simulink library "FuelSystemLibrary"  (R2014b)
settings: Solver=ode45  SolverMode=SingleTasking  StartTime=0.0  StopTime=10.0  RelTol=1e-3
undefined symbols (not defined in the file): BooleanOff, BooleanOn, BoolThreshold, BowserOnPressure, CouplingOffPressure, CouplingOnPressure, DefaultTemp, DiffuserResistance, DiscreteSwitchOff, DiscreteSwitchOn, DiscreteSwitchThreshold, FloatingPressure, FlowNoOverride, FspSamplingPeriod, FuelSpecificHeatCapacity, g, InfiniteFlow, InfiniteMass, InfiniteResistance, InfiniteTime, InfiniteVolume, kpl2kpm3, MaxAValue, MaxBValue, MeterNoReset, MinAValue, MinBValue, NearZeroMass, NearZeroTime, NoError, NominalAValue, NominalBValue, NonRetResistance, NoReset, NullBasePress, PerCycle2PerSec, PerSec2PerCycle, PipeDisconnected, PipeResistance, PumpOnTime, TankFixedMassError, TankInletResistance, TankInstPortStartOffset, TankNoReset, TypicalFuelDensity, ValveClosedPosition, ValveOnResistance, ValveOpenPosition, ValveOpenTime
libraries: FuelSystemLibrary x251, WrightSolverLib x50, simulink x1
(part 3 of 4)

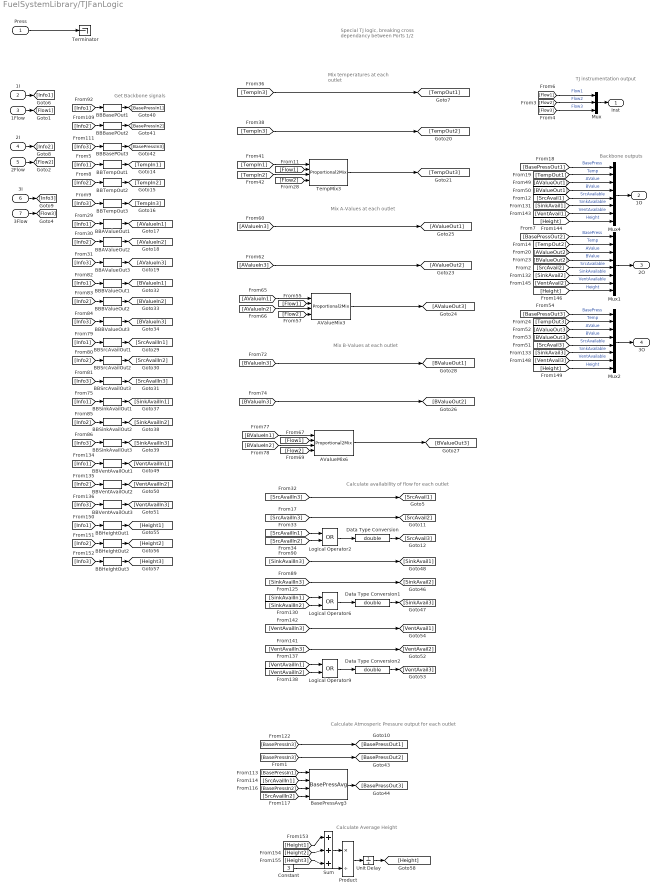
== system FuelSystemLibrary/TJFanLogic ==
  note: TJ instrumentation
      |  output
  note: Calculate availability of flow for each outlet
  note: Mix temperatures
      | at each outlet
  note: Backbone outputs
  note: Get Backbone signals
  note: Mix A-Values at each outlet
  note: Mix B-Values at each outlet
  note: Calculate Atmosperic Pressure output for each outlet
  note: Special TJ logic, breaking
      | cross dependancy
      | between Ports 1/2
  note: Calculate Average Height
  Press : Inport
  1I : Inport  Port=2
  1Flow : Inport  Port=3
  2I : Inport  Port=4
  2Flow : Inport  Port=5
  3I : Inport  Port=6
  3Flow : Inport  Port=7
  AValueMix3 : FuelSystemLibrary/Proportional2Mix
  AValueMix6 : FuelSystemLibrary/Proportional2Mix
  BBAValueOut1 : FuelSystemLibrary/BBAValueOut
  BBAValueOut2 : FuelSystemLibrary/BBAValueOut
  BBAValueOut3 : FuelSystemLibrary/BBAValueOut
  BBBValueOut1 : FuelSystemLibrary/BBBValueOut
  BBBValueOut2 : FuelSystemLibrary/BBBValueOut
  BBBValueOut3 : FuelSystemLibrary/BBBValueOut
  BBBasePOut1 : FuelSystemLibrary/BBBasePOut
  BBBasePOut2 : FuelSystemLibrary/BBBasePOut
  BBBasePOut3 : FuelSystemLibrary/BBBasePOut
  BBHeightOut1 : FuelSystemLibrary/BBHeightOut
  BBHeightOut2 : FuelSystemLibrary/BBHeightOut
  BBHeightOut3 : FuelSystemLibrary/BBHeightOut
  BBSinkAvailOut1 : FuelSystemLibrary/BBSinkAvailOut
  BBSinkAvailOut2 : FuelSystemLibrary/BBSinkAvailOut
  BBSinkAvailOut3 : FuelSystemLibrary/BBSinkAvailOut
  BBSrcAvailOut1 : FuelSystemLibrary/BBSrcAvailOut
  BBSrcAvailOut2 : FuelSystemLibrary/BBSrcAvailOut
  BBSrcAvailOut3 : FuelSystemLibrary/BBSrcAvailOut
  BBTempOut1 : FuelSystemLibrary/BBTempOut
  BBTempOut2 : FuelSystemLibrary/BBTempOut
  BBTempOut3 : FuelSystemLibrary/BBTempOut
  BBVentAvailOut1 : FuelSystemLibrary/BBVentAvailOut
  BBVentAvailOut2 : FuelSystemLibrary/BBVentAvailOut
  BBVentAvailOut3 : FuelSystemLibrary/BBVentAvailOut
  BasePressAvg3 : FuelSystemLibrary/BasePressAvg
  Constant : Constant  Value=3
  Data Type Conversion : DataTypeConversion  OutDataTypeStr=double
  Data Type Conversion1 : DataTypeConversion  OutDataTypeStr=double
  Data Type Conversion2 : DataTypeConversion  OutDataTypeStr=double
  Logical Operator2 : Logic  Operator=OR  AllPortsSameDT=off
  Logical Operator6 : Logic  Operator=OR  AllPortsSameDT=off
  Logical Operator9 : Logic  Operator=OR  AllPortsSameDT=off
  Mux : Mux  Inputs=[1 1 1]
  Mux1 : Mux  Inputs=8
  Mux2 : Mux  Inputs=8
  Mux4 : Mux  Inputs=8
  Product : Product  Inputs=*/  SaturateOnIntegerOverflow=on  InputSameDT=on  OutDataTypeStr=Inherit: Same as first input
  Sum : Sum  Inputs=|+++  SaturateOnIntegerOverflow=on  InputSameDT=on  OutDataTypeStr=Inherit: Same as first input
  TempMix3 : FuelSystemLibrary/Proportional2Mix
  Terminator : Terminator
  Unit Delay : UnitDelay  SampleTime=FspSamplingPeriod
  Inst : Outport
  1O : Outport  Port=2
  2O : Outport  Port=3
  3O : Outport  Port=4
  wires:
  1I/1 -> [Info1]
  1Flow/1 -> [Flow1]
  2Flow/1 -> [Flow2]
  3I/1 -> [Info3]
  3Flow/1 -> [Flow3]
  2I/1 -> [Info2]
  [Flow2] -> Mux/2  "Flow2"
  [Flow1] -> Mux/1  "Flow1"
  [Flow3] -> Mux/3  "Flow3"
  [Info1] -> BBTempOut1/1
  [Info2] -> BBTempOut2/1
  [Info3] -> BBTempOut3/1
  [Flow2] -> TempMix3/4
  BBTempOut1/1 -> [TempIn1]
  BBTempOut2/1 -> [TempIn2]
  BBTempOut3/1 -> [TempIn3]
  [Info1] -> BBAValueOut1/1
  [Info2] -> BBAValueOut2/1
  [Info3] -> BBAValueOut3/1
  [SrcAvailIn3] -> [SrcAvail1]
  [SrcAvailIn3] -> [SrcAvail2]
  [SrcAvailIn1] -> Logical Operator2/1
  [SrcAvailIn2] -> Logical Operator2/2
  Logical Operator2/1 -> Data Type Conversion/1
  [TempIn3] -> [TempOut1]
  [TempIn3] -> [TempOut2]
  [TempIn1] -> TempMix3/1
  [TempIn2] -> TempMix3/3
  [Flow1] -> TempMix3/2
  [SrcAvail1] -> Mux4/5  "SrcAvailable"
  [TempOut1] -> Mux4/2  "Temp"
  [BasePressOut1] -> Mux4/1  "BasePress"
  [AValueOut1] -> Mux4/3  "AValue"
  [BValueOut1] -> Mux4/4  "BValue"
  Mux4/1 -> 1O/1
  [SrcAvail2] -> Mux1/5  "SrcAvailable"
  [TempOut2] -> Mux1/2  "Temp"
  [BasePressOut2] -> Mux1/1  "BasePress"
  [AValueOut2] -> Mux1/3  "AValue"
  [BValueOut2] -> Mux1/4  "BValue"
  Mux1/1 -> 2O/1
  [SrcAvail3] -> Mux2/5  "SrcAvailable"
  [TempOut3] -> Mux2/2  "Temp"
  [BasePressOut3] -> Mux2/1  "BasePress"
  [AValueOut3] -> Mux2/3  "AValue"
  [BValueOut3] -> Mux2/4  "BValue"
  [Flow2] -> AValueMix3/4
  [AValueIn3] -> [AValueOut1]
  [AValueIn3] -> [AValueOut2]
  [AValueIn1] -> AValueMix3/1
  [AValueIn2] -> AValueMix3/3
  AValueMix3/1 -> [AValueOut3]
  [Flow1] -> AValueMix3/2
  [Flow2] -> AValueMix6/4
  [BValueIn3] -> [BValueOut1]
  [BValueIn3] -> [BValueOut2]
  [BValueIn1] -> AValueMix6/1
  [BValueIn2] -> AValueMix6/3
  AValueMix6/1 -> [BValueOut3]
  [Flow1] -> AValueMix6/2
  [Info1] -> BBSrcAvailOut1/1
  [Info2] -> BBSrcAvailOut2/1
  [Info3] -> BBSrcAvailOut3/1
  BBSrcAvailOut1/1 -> [SrcAvailIn1]
  BBSrcAvailOut2/1 -> [SrcAvailIn2]
  BBSrcAvailOut3/1 -> [SrcAvailIn3]
  BBAValueOut1/1 -> [AValueIn1]
  BBAValueOut2/1 -> [AValueIn2]
  BBAValueOut3/1 -> [AValueIn3]
  [Info1] -> BBBValueOut1/1
  [Info2] -> BBBValueOut2/1
  [Info3] -> BBBValueOut3/1
  BBBValueOut1/1 -> [BValueIn1]
  BBBValueOut2/1 -> [BValueIn2]
  BBBValueOut3/1 -> [BValueIn3]
  TempMix3/1 -> [TempOut3]
  Press/1 -> Terminator/1
  [Info1] -> BBBasePOut1/1
  BBBasePOut1/1 -> [BasePressIn1]
  [Info2] -> BBBasePOut2/1
  [Info3] -> BBBasePOut3/1
  BBBasePOut2/1 -> [BasePressIn2]
  BBBasePOut3/1 -> [BasePressIn3]
  [BasePressIn3] -> [BasePressOut1]
  [BasePressIn3] -> [BasePressOut2]
  [BasePressIn1] -> BasePressAvg3/1
  [SrcAvailIn1] -> BasePressAvg3/2
  [BasePressIn2] -> BasePressAvg3/3
  [SrcAvailIn2] -> BasePressAvg3/4
  BasePressAvg3/1 -> [BasePressOut3]
  [Info1] -> BBSinkAvailOut1/1
  BBSinkAvailOut1/1 -> [SinkAvailIn1]
  [Info2] -> BBSinkAvailOut2/1
  BBSinkAvailOut2/1 -> [SinkAvailIn2]
  [Info3] -> BBSinkAvailOut3/1
  BBSinkAvailOut3/1 -> [SinkAvailIn3]
  [SinkAvailIn3] -> [SinkAvail1]
  [SinkAvailIn3] -> [SinkAvail2]
  [SinkAvailIn1] -> Logical Operator6/1
  [SinkAvailIn2] -> Logical Operator6/2
  Logical Operator6/1 -> Data Type Conversion1/1
  [SinkAvail1] -> Mux4/6  "SinkAvailable"
  [SinkAvail2] -> Mux1/6  "SinkAvailable"
  [SinkAvail3] -> Mux2/6  "SinkAvailable"
  [Info1] -> BBVentAvailOut1/1
  BBVentAvailOut1/1 -> [VentAvailIn1]
  [Info2] -> BBVentAvailOut2/1
  BBVentAvailOut2/1 -> [VentAvailIn2]
  [Info3] -> BBVentAvailOut3/1
  BBVentAvailOut3/1 -> [VentAvailIn3]
  [VentAvailIn3] -> [VentAvail1]
  [VentAvailIn3] -> [VentAvail2]
  [VentAvailIn1] -> Logical Operator9/1
  [VentAvailIn2] -> Logical Operator9/2
  Logical Operator9/1 -> Data Type Conversion2/1
  [VentAvail1] -> Mux4/7  "VentAvailable"
  [Height] -> Mux4/8  "Height"
  [VentAvail2] -> Mux1/7  "VentAvailable"
  [Height] -> Mux1/8  "Height"
  Mux2/1 -> 3O/1
  [VentAvail3] -> Mux2/7  "VentAvailable"
  [Height] -> Mux2/8  "Height"
  [Info1] -> BBHeightOut1/1
  BBHeightOut1/1 -> [Height1]
  [Info2] -> BBHeightOut2/1
  BBHeightOut2/1 -> [Height2]
  [Info3] -> BBHeightOut3/1
  BBHeightOut3/1 -> [Height3]
  Mux/1 -> Inst/1
  Data Type Conversion/1 -> [SrcAvail3]
  Data Type Conversion1/1 -> [SinkAvail3]
  Data Type Conversion2/1 -> [VentAvail3]
  [Height1] -> Sum/1
  [Height2] -> Sum/2
  [Height3] -> Sum/3
  Sum/1 -> Product/1
  Product/1 -> Unit Delay/1
  Constant/1 -> Product/2
  Unit Delay/1 -> [Height]

== system FuelSystemLibrary/TJIntersect ==
  note: TJNet2I10 - Block to model T-junction behaviour - currently "perfect" connection
      |
      | Revision History -
      | Issue 1.0 - ?? - SW - Initial Issue
      | Issue 1.1 - 28th October 2005 - DR - Added to FSP Generic Library
  TJ : WrightSolverLib/TJ
  1P : PMIOPort  Tag=PMCPort  Port=1  Side=Left
  2P : PMIOPort  Tag=PMCPort  Port=2  Side=Left
  3P : PMIOPort  Tag=PMCPort  Port=3  Side=Right
  connections:
  1P/RConn1 -- TJ/LConn1
  TJ/RConn1 -- 3P/RConn1
  2P/RConn1 -- TJ/RConn2

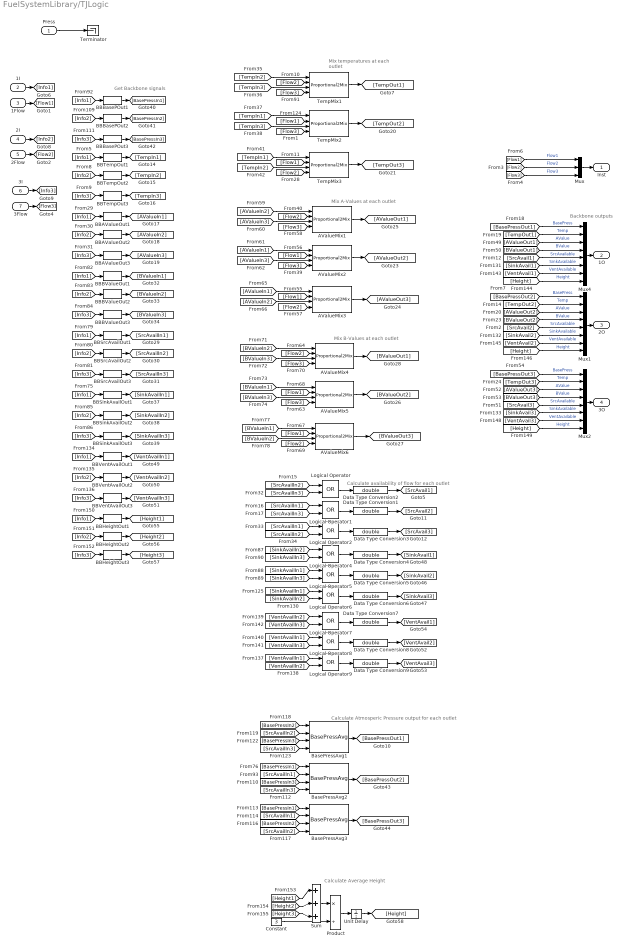
== system FuelSystemLibrary/TJLogic ==
  note: Backbone outputs
  note: Get Backbone signals
  note: Calculate Average Height
  note: Mix B-Values at each outlet
  note: Mix A-Values at each outlet
  note: Mix temperatures
      | at each outlet
  note: Calculate availability of flow for each outlet
  note: Calculate Atmosperic Pressure output for each outlet
  Press : Inport
  1I : Inport  Port=2
  1Flow : Inport  Port=3
  2I : Inport  Port=4
  2Flow : Inport  Port=5
  3I : Inport  Port=6
  3Flow : Inport  Port=7
  AValueMix{1..6} (6 alike) : FuelSystemLibrary/Proportional2Mix
  BBAValueOut1 : FuelSystemLibrary/BBAValueOut
  BBAValueOut2 : FuelSystemLibrary/BBAValueOut
  BBAValueOut3 : FuelSystemLibrary/BBAValueOut
  BBBValueOut1 : FuelSystemLibrary/BBBValueOut
  BBBValueOut2 : FuelSystemLibrary/BBBValueOut
  BBBValueOut3 : FuelSystemLibrary/BBBValueOut
  BBBasePOut1 : FuelSystemLibrary/BBBasePOut
  BBBasePOut2 : FuelSystemLibrary/BBBasePOut
  BBBasePOut3 : FuelSystemLibrary/BBBasePOut
  BBHeightOut1 : FuelSystemLibrary/BBHeightOut
  BBHeightOut2 : FuelSystemLibrary/BBHeightOut
  BBHeightOut3 : FuelSystemLibrary/BBHeightOut
  BBSinkAvailOut1 : FuelSystemLibrary/BBSinkAvailOut
  BBSinkAvailOut2 : FuelSystemLibrary/BBSinkAvailOut
  BBSinkAvailOut3 : FuelSystemLibrary/BBSinkAvailOut
  BBSrcAvailOut1 : FuelSystemLibrary/BBSrcAvailOut
  BBSrcAvailOut2 : FuelSystemLibrary/BBSrcAvailOut
  BBSrcAvailOut3 : FuelSystemLibrary/BBSrcAvailOut
  BBTempOut1 : FuelSystemLibrary/BBTempOut
  BBTempOut2 : FuelSystemLibrary/BBTempOut
  BBTempOut3 : FuelSystemLibrary/BBTempOut
  BBVentAvailOut1 : FuelSystemLibrary/BBVentAvailOut
  BBVentAvailOut2 : FuelSystemLibrary/BBVentAvailOut
  BBVentAvailOut3 : FuelSystemLibrary/BBVentAvailOut
  BasePressAvg1 : FuelSystemLibrary/BasePressAvg
  BasePressAvg2 : FuelSystemLibrary/BasePressAvg
  BasePressAvg3 : FuelSystemLibrary/BasePressAvg
  Constant : Constant  Value=3
  Data Type Conversion{1..9} (9 alike) : DataTypeConversion  OutDataTypeStr=double
  Logical Operator{,1..2,4..9} (9 alike) : Logic  Operator=OR  AllPortsSameDT=off
  Mux : Mux  Inputs=[1 1 1]
  Mux1 : Mux  Inputs=8
  Mux2 : Mux  Inputs=8
  Mux4 : Mux  Inputs=8
  Product : Product  Inputs=*/  SaturateOnIntegerOverflow=on  InputSameDT=on  OutDataTypeStr=Inherit: Same as first input
  Sum : Sum  Inputs=|+++  SaturateOnIntegerOverflow=on  InputSameDT=on  OutDataTypeStr=Inherit: Same as first input
  TempMix1 : FuelSystemLibrary/Proportional2Mix
  TempMix2 : FuelSystemLibrary/Proportional2Mix
  TempMix3 : FuelSystemLibrary/Proportional2Mix
  Terminator : Terminator
  Unit Delay : UnitDelay  SampleTime=FspSamplingPeriod
  Inst : Outport
  1O : Outport  Port=2
  2O : Outport  Port=3
  3O : Outport  Port=4
  wires:
  1I/1 -> [Info1]
  1Flow/1 -> [Flow1]
  2Flow/1 -> [Flow2]
  3I/1 -> [Info3]
  3Flow/1 -> [Flow3]
  2I/1 -> [Info2]
  [Flow2] -> Mux/2  "Flow2"
  [Flow1] -> Mux/1  "Flow1"
  [Flow3] -> Mux/3  "Flow3"
  [Info1] -> BBTempOut1/1
  [Info2] -> BBTempOut2/1
  [Info3] -> BBTempOut3/1
  BBTempOut1/1 -> [TempIn1]
  BBTempOut2/1 -> [TempIn2]
  BBTempOut3/1 -> [TempIn3]
  [Info1] -> BBAValueOut1/1
  [Info2] -> BBAValueOut2/1
  [Info3] -> BBAValueOut3/1
  [SrcAvail1] -> Mux4/5  "SrcAvailable"
  [TempOut1] -> Mux4/2  "Temp"
  [BasePressOut1] -> Mux4/1  "BasePress"
  [AValueOut1] -> Mux4/3  "AValue"
  [BValueOut1] -> Mux4/4  "BValue"
  [SrcAvail2] -> Mux1/5  "SrcAvailable"
  [TempOut2] -> Mux1/2  "Temp"
  [BasePressOut2] -> Mux1/1  "BasePress"
  [AValueOut2] -> Mux1/3  "AValue"
  [BValueOut2] -> Mux1/4  "BValue"
  [SrcAvail3] -> Mux2/5  "SrcAvailable"
  [TempOut3] -> Mux2/2  "Temp"
  [BasePressOut3] -> Mux2/1  "BasePress"
  [AValueOut3] -> Mux2/3  "AValue"
  [BValueOut3] -> Mux2/4  "BValue"
  [Info1] -> BBSrcAvailOut1/1
  [Info2] -> BBSrcAvailOut2/1
  [Info3] -> BBSrcAvailOut3/1
  BBSrcAvailOut1/1 -> [SrcAvailIn1]
  BBSrcAvailOut2/1 -> [SrcAvailIn2]
  BBSrcAvailOut3/1 -> [SrcAvailIn3]
  BBAValueOut1/1 -> [AValueIn1]
  BBAValueOut2/1 -> [AValueIn2]
  BBAValueOut3/1 -> [AValueIn3]
  [Info1] -> BBBValueOut1/1
  [Info2] -> BBBValueOut2/1
  [Info3] -> BBBValueOut3/1
  BBBValueOut1/1 -> [BValueIn1]
  BBBValueOut2/1 -> [BValueIn2]
  BBBValueOut3/1 -> [BValueIn3]
  [Info1] -> BBBasePOut1/1
  BBBasePOut1/1 -> [BasePressIn1]
  [Info2] -> BBBasePOut2/1
  [Info3] -> BBBasePOut3/1
  Press/1 -> Terminator/1
  BBBasePOut2/1 -> [BasePressIn2]
  BBBasePOut3/1 -> [BasePressIn3]
  [Info1] -> BBSinkAvailOut1/1
  BBSinkAvailOut1/1 -> [SinkAvailIn1]
  [Info2] -> BBSinkAvailOut2/1
  BBSinkAvailOut2/1 -> [SinkAvailIn2]
  [Info3] -> BBSinkAvailOut3/1
  BBSinkAvailOut3/1 -> [SinkAvailIn3]
  [SinkAvail1] -> Mux4/6  "SinkAvailable"
  [SinkAvail2] -> Mux1/6  "SinkAvailable"
  [SinkAvail3] -> Mux2/6  "SinkAvailable"
  [Info1] -> BBVentAvailOut1/1
  BBVentAvailOut1/1 -> [VentAvailIn1]
  [Info2] -> BBVentAvailOut2/1
  BBVentAvailOut2/1 -> [VentAvailIn2]
  [Info3] -> BBVentAvailOut3/1
  BBVentAvailOut3/1 -> [VentAvailIn3]
  [VentAvail1] -> Mux4/7  "VentAvailable"
  [Height] -> Mux4/8  "Height"
  [VentAvail2] -> Mux1/7  "VentAvailable"
  [Height] -> Mux1/8  "Height"
  [VentAvail3] -> Mux2/7  "VentAvailable"
  [Height] -> Mux2/8  "Height"
  [Info1] -> BBHeightOut1/1
  BBHeightOut1/1 -> [Height1]
  [Info2] -> BBHeightOut2/1
  BBHeightOut2/1 -> [Height2]
  [Info3] -> BBHeightOut3/1
  BBHeightOut3/1 -> [Height3]
  Mux/1 -> Inst/1
  Mux1/1 -> 2O/1
  Mux2/1 -> 3O/1
  Mux4/1 -> 1O/1
  [SrcAvailIn2] -> Logical Operator/1
  Logical Operator/1 -> Data Type Conversion2/1
  [Flow1] -> TempMix2/2
  [Flow3] -> TempMix2/4
  [Flow2] -> TempMix3/4
  [Flow3] -> TempMix1/4
  [Flow2] -> TempMix1/2
  [SrcAvailIn3] -> Logical Operator/2
  [SrcAvailIn1] -> Logical Operator1/1
  [SrcAvailIn3] -> Logical Operator1/2
  Logical Operator1/1 -> Data Type Conversion1/1
  [SrcAvailIn1] -> Logical Operator2/1
  [SrcAvailIn2] -> Logical Operator2/2
  Logical Operator2/1 -> Data Type Conversion3/1
  [TempIn2] -> TempMix1/1
  [TempIn3] -> TempMix1/3
  [TempIn1] -> TempMix2/1
  [TempIn3] -> TempMix2/3
  [TempIn1] -> TempMix3/1
  [TempIn2] -> TempMix3/3
  [Flow1] -> TempMix3/2
  AValueMix1/1 -> [AValueOut1]
  [Flow1] -> AValueMix2/2
  [Flow3] -> AValueMix2/4
  [Flow2] -> AValueMix3/4
  [Flow2] -> AValueMix1/2
  [AValueIn2] -> AValueMix1/1
  [AValueIn3] -> AValueMix1/3
  [AValueIn1] -> AValueMix2/1
  [AValueIn3] -> AValueMix2/3
  [AValueIn1] -> AValueMix3/1
  [AValueIn2] -> AValueMix3/3
  AValueMix2/1 -> [AValueOut2]
  AValueMix3/1 -> [AValueOut3]
  [Flow1] -> AValueMix3/2
  AValueMix4/1 -> [BValueOut1]
  [Flow1] -> AValueMix5/2
  [Flow3] -> AValueMix5/4
  [Flow2] -> AValueMix6/4
  [Flow3] -> AValueMix4/4
  [Flow2] -> AValueMix4/2
  [BValueIn2] -> AValueMix4/1
  [BValueIn3] -> AValueMix4/3
  [BValueIn1] -> AValueMix5/1
  [BValueIn3] -> AValueMix5/3
  [BValueIn1] -> AValueMix6/1
  [BValueIn2] -> AValueMix6/3
  AValueMix5/1 -> [BValueOut2]
  AValueMix6/1 -> [BValueOut3]
  [Flow1] -> AValueMix6/2
  TempMix1/1 -> [TempOut1]
  TempMix2/1 -> [TempOut2]
  TempMix3/1 -> [TempOut3]
  [Flow3] -> AValueMix1/4
  [SinkAvailIn2] -> Logical Operator4/1
  Logical Operator4/1 -> Data Type Conversion4/1
  [SinkAvailIn3] -> Logical Operator4/2
  [SinkAvailIn1] -> Logical Operator5/1
  [SinkAvailIn3] -> Logical Operator5/2
  Logical Operator5/1 -> Data Type Conversion5/1
  [SinkAvailIn1] -> Logical Operator6/1
  [SinkAvailIn2] -> Logical Operator6/2
  Logical Operator6/1 -> Data Type Conversion6/1
  [VentAvailIn2] -> Logical Operator7/1
  Logical Operator7/1 -> Data Type Conversion7/1
  [VentAvailIn3] -> Logical Operator7/2
  [VentAvailIn1] -> Logical Operator8/1
  [VentAvailIn3] -> Logical Operator8/2
  Logical Operator8/1 -> Data Type Conversion8/1
  [VentAvailIn1] -> Logical Operator9/1
  [VentAvailIn2] -> Logical Operator9/2
  Logical Operator9/1 -> Data Type Conversion9/1
  [Height1] -> Sum/1
  [Height2] -> Sum/2
  [Height3] -> Sum/3
  Sum/1 -> Product/1
  Product/1 -> Unit Delay/1
  Constant/1 -> Product/2
  Unit Delay/1 -> [Height]
  [BasePressIn2] -> BasePressAvg1/1
  [SrcAvailIn2] -> BasePressAvg1/2
  [BasePressIn3] -> BasePressAvg1/3
  [SrcAvailIn3] -> BasePressAvg1/4
  BasePressAvg1/1 -> [BasePressOut1]
  [BasePressIn1] -> BasePressAvg2/1
  [SrcAvailIn1] -> BasePressAvg2/2
  [BasePressIn3] -> BasePressAvg2/3
  [SrcAvailIn3] -> BasePressAvg2/4
  BasePressAvg2/1 -> [BasePressOut2]
  [BasePressIn1] -> BasePressAvg3/1
  [SrcAvailIn1] -> BasePressAvg3/2
  [BasePressIn2] -> BasePressAvg3/3
  [SrcAvailIn2] -> BasePressAvg3/4
  BasePressAvg3/1 -> [BasePressOut3]
  Data Type Conversion2/1 -> [SrcAvail1]
  Data Type Conversion1/1 -> [SrcAvail2]
  Data Type Conversion3/1 -> [SrcAvail3]
  Data Type Conversion4/1 -> [SinkAvail1]
  Data Type Conversion5/1 -> [SinkAvail2]
  Data Type Conversion6/1 -> [SinkAvail3]
  Data Type Conversion7/1 -> [VentAvail1]
  Data Type Conversion8/1 -> [VentAvail2]
  Data Type Conversion9/1 -> [VentAvail3]

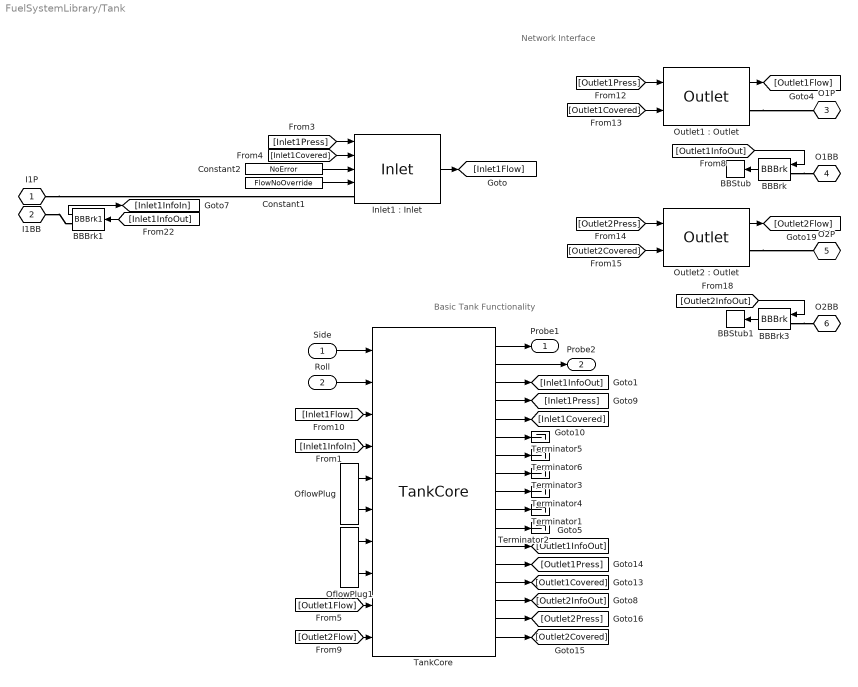
== system FuelSystemLibrary/Tank ==
  note: Network Interface
  note: Basic Tank Functionality
  Side : Inport
  Roll : Inport  Port=2
  BBBrk : FuelSystemLibrary/BBBrk
  BBBrk1 : FuelSystemLibrary/BBBrk1
  BBBrk3 : FuelSystemLibrary/BBBrk
  BBStub : FuelSystemLibrary/BBStub
  BBStub1 : FuelSystemLibrary/BBStub
  Constant1 : Constant  Value=FlowNoOverride
  Constant2 : Constant  Value=NoError
  "Inlet1 : Inlet" : FuelSystemLibrary/Inlet  TankInletResistance=TankInletResistance
  OflowPlug : FuelSystemLibrary/OflowPlug
  OflowPlug1 : FuelSystemLibrary/OflowPlug
  "Outlet1 : Outlet" : FuelSystemLibrary/Outlet
  "Outlet2 : Outlet" : FuelSystemLibrary/Outlet
  TankCore : FuelSystemLibrary/TankCore
  Terminator{1..6} (6 alike) : Terminator
  I1P : PMIOPort  Tag=PMCPort  Port=1  Side=Left
  I1BB : PMIOPort  Tag=PMCPort  Port=2  Side=Left
  O1P : PMIOPort  Tag=PMCPort  Port=3  Side=Right
  O1BB : PMIOPort  Tag=PMCPort  Port=4  Side=Right
  O2P : PMIOPort  Tag=PMCPort  Port=5  Side=Right
  O2BB : PMIOPort  Tag=PMCPort  Port=6  Side=Right
  Probe1 : Outport
  Probe2 : Outport  Port=2
  wires:
  [Outlet2InfoOut] -> BBBrk3/1
  BBBrk3/1 -> BBStub1/1
  BBBrk/1 -> BBStub/1
  "Outlet2 : Outlet"/1 -> [Outlet2Flow]
  "Inlet1 : Inlet"/1 -> [Inlet1Flow]
  BBBrk1/1 -> [Inlet1InfoIn]
  [Inlet1InfoOut] -> BBBrk1/1
  "Outlet1 : Outlet"/1 -> [Outlet1Flow]
  TankCore/2 -> Probe2/1
  TankCore/1 -> Probe1/1
  [Inlet1InfoIn] -> TankCore/4
  OflowPlug/2 -> TankCore/6
  [Inlet1Press] -> "Inlet1 : Inlet"/1
  [Inlet1Covered] -> "Inlet1 : Inlet"/2
  [Inlet1Flow] -> TankCore/3
  OflowPlug/1 -> TankCore/5
  [Outlet1Press] -> "Outlet1 : Outlet"/1
  [Outlet1Covered] -> "Outlet1 : Outlet"/2
  [Outlet2Press] -> "Outlet2 : Outlet"/1
  [Outlet2Covered] -> "Outlet2 : Outlet"/2
  [Outlet1Flow] -> TankCore/9
  [Outlet2Flow] -> TankCore/10
  [Outlet1InfoOut] -> BBBrk/1
  OflowPlug1/1 -> TankCore/7
  OflowPlug1/2 -> TankCore/8
  Constant2/1 -> "Inlet1 : Inlet"/3
  Constant1/1 -> "Inlet1 : Inlet"/4
  Roll/1 -> TankCore/2
  Side/1 -> TankCore/1
  TankCore/17 -> [Outlet2Covered]
  TankCore/3 -> [Inlet1InfoOut]
  TankCore/10 -> Terminator1/1
  TankCore/16 -> [Outlet2Press]
  TankCore/7 -> Terminator6/1
  TankCore/5 -> [Inlet1Covered]
  TankCore/8 -> Terminator3/1
  TankCore/6 -> Terminator5/1
  TankCore/4 -> [Inlet1Press]
  TankCore/11 -> Terminator2/1
  TankCore/13 -> [Outlet1Press]
  TankCore/9 -> Terminator4/1
  TankCore/14 -> [Outlet1Covered]
  TankCore/15 -> [Outlet2InfoOut]
  TankCore/12 -> [Outlet1InfoOut]
  connections:
  BBBrk3/LConn1 -- O2BB/RConn1
  BBBrk/LConn1 -- O1BB/RConn1
  "Outlet2 : Outlet"/RConn1 -- O2P/RConn1
  "Outlet1 : Outlet"/RConn1 -- O1P/RConn1
  I1P/RConn1 -- "Inlet1 : Inlet"/LConn1
  I1BB/RConn1 -- BBBrk1/RConn1

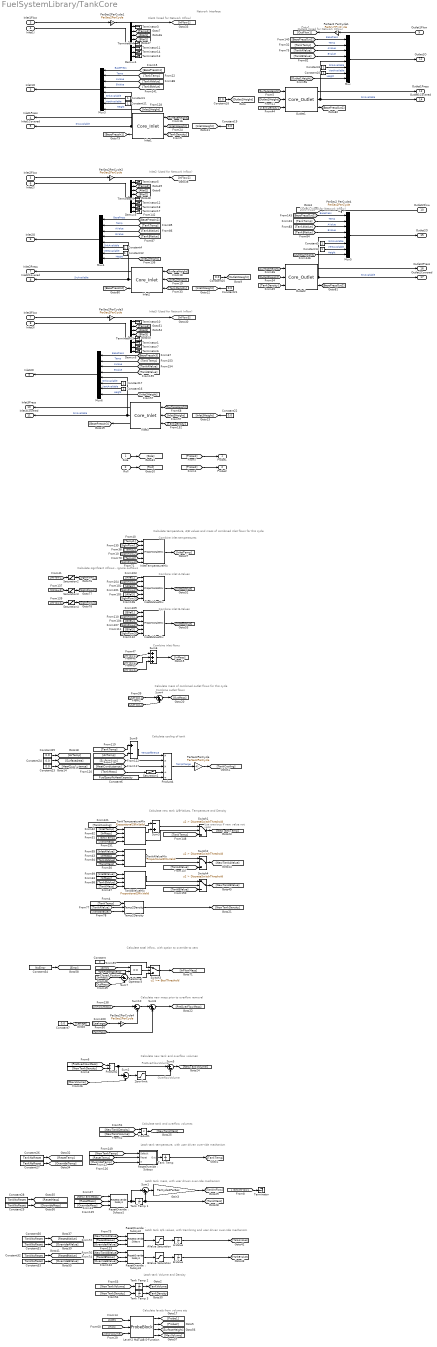
== system FuelSystemLibrary/TankCore ==
  note: Inlet3 (Used for Network Inflow)
  note: Use previous if new
      | value not valid
  note: Calculate tank and overflow volumes
  note: PreOverFlowVolume
  note: Combine inlet temperatures
  note: Combine inlet flows
  note: Latch tank mass, with user driven over-ride mechanism
  note: OverflowVolume
  note: Calculate new tank and overflow volumes
  note: Calculate new tank A/B-Values, Temperature and Density
  note: Calculate mass of combined outlet flows for this cycle
  note: Calculate temperature, A/B values and mass of combined inlet flows for this cycle
  note: Combine outlet flows
  note: Latch tank temperature, with user driven over-ride mechanism
  note: Network Interface
  note: Calculate levels from volume etc
  note: Inlet1 (Used for Network Inflow)
  note: Inlet2 (Used for Network Inflow)
  note: Outlet1 (Used for Network Inflow)
  note: Outlet2 (Used for Network Inflow)
  note: Latch tank A/b values, with tramlining and user driven over-ride mechanism
  note: Latch tank Volume and Density
  note: Calculate new mass prior to overflow removal
  note: Combine inlet A-Values
  note: Combine inlet B-Values
  note: Calculate cooling of tank
  note: Calculate significant inflows - ignore outflows
  note: Calculate total inflow, with option to override to zero
  Side : Inport
  Roll : Inport  Port=2
  Inlet1Flow : Inport  Port=3
  Inlet1I : Inport  Port=4
  Inlet2Flow : Inport  Port=5
  Inlet2I : Inport  Port=6
  Inlet3Flow : Inport  Port=7
  Inlet3I : Inport  Port=8
  Outlet1Flow : Inport  Port=9
  Outlet2Flow : Inport  Port=10
  A-Value : UnitDelay  InitialCondition=NominalAValue  SampleTime=FspSamplingPeriod
  AValue Saturation : Saturate  UpperLimit=MaxAValue  LowerLimit=MinAValue
  B-Value : UnitDelay  InitialCondition=NominalBValue  SampleTime=FspSamplingPeriod
  BValue Saturation : Saturate  UpperLimit=MaxBValue  LowerLimit=MinBValue
  Closed Position : Constant  Value=TankFixedMassError
  Constant : Constant  Value=0
  Constant{1,3..5,10..13,16..17} (10 alike) : Constant
  Constant{7,18..25} (9 alike) : Constant  Value=0.0
  Constant{26..33} (8 alike) : Constant  Value=TankNoReset
  Constant34 : Constant  Value=NoError
  Constant6 : Constant  Value=FuelSpecificHeatCapacity
  Demux4 : Demux  Outputs=8
  Demux5 : Demux  Outputs=8
  Demux6 : Demux  Outputs=8
  Gain3 : Gain  Gain=PerCycle2PerSec  OutDataTypeStr=Inherit: Same as input  ParamDataTypeStr=Inherit: Same as input
  Inlet1 : FuelSystemLibrary/Core_Inlet
  Inlet2 : FuelSystemLibrary/Core_Inlet
  Inlet3 : FuelSystemLibrary/Core_Inlet
  InletAValueMix : FuelSystemLibrary/Proportional3Mix
  InletBValueMix : FuelSystemLibrary/Proportional3Mix
  InletTemperatureMix : FuelSystemLibrary/Proportional3Mix
  Level-2 MATLAB S-Function : M-S-Function  FunctionName=ProbeBlock
  Mux{,3..6} (5 alike) : Mux  Inputs=8
  Outlet1 : FuelSystemLibrary/Core_Outlet
  Outlet2 : FuelSystemLibrary/Core_Outlet
  PerSec2 PerCycle1 : Gain  Gain=PerSec2PerCycle  OutDataTypeStr=Inherit: Same as input  ParamDataTypeStr=Inherit: Same as input
  PerSec2 PerCycle4 : Gain  Gain=PerSec2PerCycle  OutDataTypeStr=Inherit: Same as input  ParamDataTypeStr=Inherit: Same as input
  PerSec2PerCycle{,1..4} (5 alike) : Gain  Gain=PerSec2PerCycle  OutDataTypeStr=Inherit: Same as input  ParamDataTypeStr=Inherit: Same as input
  Product1 : Product  SaturateOnIntegerOverflow=on  InputSameDT=on  OutDataTypeStr=Inherit: Same as first input
  Product2 : Product  Inputs=*/  SaturateOnIntegerOverflow=on  InputSameDT=on  OutDataTypeStr=Inherit: Same as first input
  Product4 : Product  Inputs=***//  SaturateOnIntegerOverflow=on  OutDataTypeStr=Inherit: Same as first input
  Relational Operator3 : RelationalOperator  Operator===  ZeroCross=off
  "ResetOveride : Subsys" : Subsystem
  "ResetOveride : Subsys1" : FuelSystemLibrary/TankCore/ResetOveride :  Subsys
  "ResetOveride : Subsys2" : FuelSystemLibrary/TankCore/ResetOveride :  Subsys
  "ResetOveride : Subsys3" : FuelSystemLibrary/TankCore/ResetOveride :  Subsys
  Saturation1 : Saturate  UpperLimit=InfiniteMass  LowerLimit=NearZeroMass
  Saturation2 : Saturate  UpperLimit=InfiniteFlow  LowerLimit=0
  Saturation3 : Saturate  UpperLimit=InfiniteFlow  LowerLimit=0
  Saturation4 : Saturate  UpperLimit=InfiniteFlow  LowerLimit=0
  Sum{1..2,5,7,9..10} (6 alike) : Sum  Inputs=|+-  SaturateOnIntegerOverflow=on  InputSameDT=on  OutDataTypeStr=Inherit: Same as first input
  Sum3 : Sum  Inputs=|-+  SaturateOnIntegerOverflow=on
  Sum4 : Sum  Inputs=|++  SaturateOnIntegerOverflow=on  InputSameDT=on  OutDataTypeStr=Inherit: Same as first input
  Sum6 : Sum  Inputs=|+++  SaturateOnIntegerOverflow=on  InputSameDT=on  OutDataTypeStr=Inherit: Same as first input
  Sum8 : Sum  Inputs=|++  SaturateOnIntegerOverflow=on  InputSameDT=on  OutDataTypeStr=Inherit: Same as first input
  Switch1 : Switch  Criteria=u2 > Threshold  Threshold=DiscreteSwitchThreshold  SaturateOnIntegerOverflow=on  InputSameDT=on
  Switch2 : Switch  Criteria=u2 > Threshold  Threshold=DiscreteSwitchThreshold  SaturateOnIntegerOverflow=on  InputSameDT=on
  Switch3 : Switch  Threshold=BoolThreshold  SaturateOnIntegerOverflow=on  InputSameDT=on
  Switch4 : Switch  Criteria=u2 > Threshold  Threshold=DiscreteSwitchThreshold  SaturateOnIntegerOverflow=on  InputSameDT=on
  "Tank Temp " : UnitDelay  InitialCondition=DefaultTemp  SampleTime=FspSamplingPeriod
  Tank Temp 1 : UnitDelay  InitialCondition=NearZeroMass  SampleTime=FspSamplingPeriod
  Tank Temp 2 : UnitDelay  SampleTime=FspSamplingPeriod
  Tank Temp 3 : UnitDelay  InitialCondition=TypicalFuelDensity  SampleTime=FspSamplingPeriod
  TankAValueMix : FuelSystemLibrary/Proportional2MixValid
  TankBValueMix : FuelSystemLibrary/Proportional2MixValid
  TankTemperatureMix : FuelSystemLibrary/Proportional2MixValid
  Temp2Density : FuelSystemLibrary/Temp2Density
  Terminator{,1,3..7,9..15,17..18} (16 alike) : Terminator
  Zero-limit : Saturate  UpperLimit=InfiniteVolume  LowerLimit=0
  Probe1 : Outport
  Probe2 : Outport  Port=2
  Inlet1O : Outport  Port=3
  Inlet1Press : Outport  Port=4
  Inlet1Covered : Outport  Port=5
  Inlet2O : Outport  Port=6
  Inlet2Press : Outport  Port=7
  Inlet2Covered : Outport  Port=8
  Inlet3O : Outport  Port=9
  Inlet3Press : Outport  Port=10
  Inlet3Covered : Outport  Port=11
  Outlet1O : Outport  Port=12
  Outlet1Press : Outport  Port=13
  Outlet1Covered : Outport  Port=14
  Outlet2O : Outport  Port=15
  Outlet2Press : Outport  Port=16
  Outlet2Covered : Outport  Port=17
  wires:
  Inlet3Flow/1 -> PerSec2PerCycle3/1
  Demux6/2 -> [Temp3]
  Demux6/1 -> Terminator10/1
  Demux6/3 -> [AVal3]
  Demux6/4 -> [BVal3]
  Demux6/5 -> Terminator15/1
  Inlet3I/1 -> Demux6/1
  PerSec2PerCycle3/1 -> [InFlow3]
  Demux6/6 -> Terminator1/1
  Demux6/7 -> Terminator7/1
  Demux6/8 -> Terminator6/1
  Inlet3/1 -> Inlet3Press/1
  Inlet3/2 -> Inlet3Covered/1, Mux6/5  "SrcAvailable"
  Mux6/1 -> Inlet3O/1
  [BasePressIn3] -> Mux6/1  "BasePress"
  [TankTemp] -> Mux6/2  "Temp"
  [TankAValue] -> Mux6/3  "AValue"
  [TankBValue] -> Mux6/4  "BValue"
  [SurfaceHeight] -> Inlet3/1
  [Inlet3Height] -> Inlet3/2
  [TankDensity] -> Inlet3/3
  Inlet3/3 -> [BasePressIn3]
  Constant17/1 -> Mux6/6  "SinkAvailable"
  [Inlet3Height] -> Mux6/8  "Height"
  Constant16/1 -> Mux6/7  "VentAvailable"
  Switch4/1 -> [NewTankBValue]
  [TankBValue] -> Switch4/3
  TankBValueMix/2 -> Switch4/2
  TankBValueMix/1 -> Switch4/1
  Switch2/1 -> [NewTankAValue]
  [TankAValue] -> Switch2/3
  [TankTemp] -> Temp2Density/1
  Switch1/1 -> [NewTankTemp]
  [TankTemp] -> Switch1/3
  [NewTankTemp] -> "ResetOveride : Subsys"/1(Default)
  TankAValueMix/2 -> Switch2/2
  TankTemperatureMix/2 -> Switch1/2
  Tank Temp 3/1 -> [TankDensity]
  [NewTankDensity] -> Tank Temp 3/1
  Tank Temp 2/1 -> [TankVolume]
  [NewTankVolume] -> Tank Temp 2/1
  [NewTankVolume] -> Product1/2
  Product1/1 -> [NewTankMass]
  [NewTankDensity] -> Product1/1
  Temp2Density/1 -> [NewTankDensity]
  [PreOverFlowMass] -> Product2/1
  [NewTankDensity] -> Product2/2
  Sum8/1 -> [PreOverFlowMass]
  [OutMass] -> Sum7/2
  [InMass] -> Sum7/1
  TankTemperatureMix/1 -> Sum3/2
  [InFlow1] -> Sum6/1
  [TankDensity] -> Outlet2/3
  [TankDensity] -> Outlet1/3
  [TankDensity] -> Inlet1/3
  Sum1/1 -> Gain3/1
  Tank Temp 1/1 -> [TankMass], Sum1/2
  "ResetOveride : Subsys1"/1 -> Sum1/1, Tank Temp 1/1
  Sum5/1 -> [NewTankVolume]
  Zero-limit/1 -> Sum5/2
  Sum2/1 -> Zero-limit/1
  [MaxVolume] -> Sum2/2
  Product2/1 -> Sum5/1, Sum2/1
  Sum4/1 -> [OutMass]
  Gain3/1 -> [TankInFlow]
  [OutFlow2] -> Sum4/2
  [OutFlow1] -> Sum4/1
  [SurfaceHeight] -> Outlet2/1
  [Outlet2Height] -> Outlet2/2
  Demux4/2 -> [Temp1]
  Demux4/1 -> Terminator3/1
  Inlet1I/1 -> Demux4/1
  Mux/1 -> Outlet1O/1
  "Tank Temp "/1 -> [TankTemp]
  Outlet1Flow/1 -> PerSec2 PerCycle1/1
  [SurfaceHeight] -> Outlet1/1
  [Outlet1Height] -> Outlet1/2
  [Probe1] -> Probe1/1
  [Inlet1Height] -> Inlet1/2
  [SurfaceHeight] -> Inlet1/1
  Inlet1Flow/1 -> PerSec2PerCycle1/1
  Inlet2Flow/1 -> PerSec2PerCycle2/1
  Inlet1/1 -> Inlet1Press/1
  Inlet1/2 -> Inlet1Covered/1, Mux3/5  "SrcAvailable"
  Inlet2/1 -> Inlet2Press/1
  Inlet2/2 -> Inlet2Covered/1, Mux4/5  "SrcAvailable"
  Outlet2Flow/1 -> PerSec2 PerCycle4/1
  Outlet1/1 -> Outlet1Press/1
  Outlet1/2 -> Mux/5, Outlet1Covered/1  "SrcAvailable"
  Outlet2/1 -> Outlet2Press/1
  Outlet2/2 -> Outlet2Covered/1, Mux5/5  "SrcAvailable"
  Sum6/1 -> [InMass]
  InletTemperatureMix/1 -> [InletTemp]
  Demux4/3 -> [AVal1]
  [InFlow2] -> Sum6/2
  [InFlow3] -> Sum6/3
  A-Value/1 -> [TankAValue]
  B-Value/1 -> [TankBValue]
  [TankAValue] -> Temp2Density/2
  [TankBValue] -> Temp2Density/3
  Demux4/4 -> [BVal1]
  Demux4/5 -> Terminator4/1
  Demux5/2 -> [Temp2]
  Demux5/1 -> Terminator5/1
  Demux5/3 -> [AVal2]
  Demux5/4 -> [BVal2]
  Demux5/5 -> Terminator9/1
  Inlet2I/1 -> Demux5/1
  [TankTemp] -> Mux5/2  "Temp"
  [BasePressOut2] -> Mux5/1  "BasePress"
  Mux5/1 -> Outlet2O/1
  [TankAValue] -> Mux5/3  "AValue"
  [TankBValue] -> Mux5/4  "BValue"
  [TankTemp] -> Mux/2  "Temp"
  [BasePressOut1] -> Mux/1  "BasePress"
  [TankAValue] -> Mux/3  "AValue"
  [TankBValue] -> Mux/4  "BValue"
  Mux4/1 -> Inlet2O/1
  [BasePressIn2] -> Mux4/1  "BasePress"
  [TankTemp] -> Mux4/2  "Temp"
  [TankAValue] -> Mux4/3  "AValue"
  [TankBValue] -> Mux4/4  "BValue"
  Mux3/1 -> Inlet1O/1
  [BasePressIn1] -> Mux3/1  "BasePress"
  [TankTemp] -> Mux3/2  "Temp"
  [TankAValue] -> Mux3/3  "AValue"
  [TankBValue] -> Mux3/4  "BValue"
  [SigInFlow3] -> InletTemperatureMix/6
  [Temp3] -> InletTemperatureMix/5
  [SigInFlow2] -> InletTemperatureMix/4
  [Temp2] -> InletTemperatureMix/3
  [SigInFlow1] -> InletTemperatureMix/2
  [Temp1] -> InletTemperatureMix/1
  [InletTemp] -> TankTemperatureMix/1
  [InMass] -> TankTemperatureMix/2
  [TankTemp] -> TankTemperatureMix/3
  [TankMass] -> TankTemperatureMix/4
  [InletAValue] -> TankAValueMix/1
  [InMass] -> TankAValueMix/2
  [TankAValue] -> TankAValueMix/3
  [TankMass] -> TankAValueMix/4
  [InletBValue] -> TankBValueMix/1
  [InMass] -> TankBValueMix/2
  [TankBValue] -> TankBValueMix/3
  [TankMass] -> TankBValueMix/4
  InletAValueMix/1 -> [InletAValue]
  [SigInFlow3] -> InletAValueMix/6
  [AVal3] -> InletAValueMix/5
  [SigInFlow2] -> InletAValueMix/4
  [AVal2] -> InletAValueMix/3
  [SigInFlow1] -> InletAValueMix/2
  [AVal1] -> InletAValueMix/1
  InletBValueMix/1 -> [InletBValue]
  [SigInFlow3] -> InletBValueMix/6
  [BVal3] -> InletBValueMix/5
  [SigInFlow2] -> InletBValueMix/4
  [BVal2] -> InletBValueMix/3
  [SigInFlow1] -> InletBValueMix/2
  [BVal1] -> InletBValueMix/1
  TankAValueMix/1 -> Switch2/1
  [HeatConductance] -> Product4/3
  Sum9/1 -> Product4/1  "TempDifference"
  [TankMass] -> Saturation1/1
  Constant6/1 -> Product4/5
  Product4/1 -> PerSec2PerCycle/1  "TempChange"
  Sum3/1 -> Switch1/1
  [SurfaceArea] -> Product4/2
  [AirTemp] -> Sum9/2
  [TankTemp] -> Sum9/1
  Saturation1/1 -> Product4/4
  [NewTankAValue] -> "ResetOveride : Subsys2"/1
  [ResetAValue] -> "ResetOveride : Subsys2"/2
  [OverrideAValue] -> "ResetOveride : Subsys2"/3
  "ResetOveride : Subsys2"/1 -> AValue Saturation/1
  [NewTankBValue] -> "ResetOveride : Subsys3"/1
  [ResetBValue] -> "ResetOveride : Subsys3"/2
  [OverrideBValue] -> "ResetOveride : Subsys3"/3
  "ResetOveride : Subsys3"/1 -> BValue Saturation/1
  [NewTankMass] -> "ResetOveride : Subsys1"/1
  [ResetMass] -> "ResetOveride : Subsys1"/2
  [OverrideMass] -> "ResetOveride : Subsys1"/3
  [ResetTemp] -> "ResetOveride : Subsys"/2(Reset)
  [OverrideTemp] -> "ResetOveride : Subsys"/3(Override)
  "ResetOveride : Subsys"/1(Out) -> "Tank Temp "/1
  PerSec2PerCycle/1 -> [TankCooling]
  PerSec2PerCycle1/1 -> [InFlow1]
  PerSec2PerCycle2/1 -> [InFlow2]
  PerSec2 PerCycle4/1 -> [OutFlow2]
  PerSec2 PerCycle1/1 -> [OutFlow1]
  Level-2 MATLAB S-Function/1 -> [Probe1]
  [SurfaceHeight] -> Inlet2/1
  [Inlet2Height] -> Inlet2/2
  [TankDensity] -> Inlet2/3
  AValue Saturation/1 -> A-Value/1
  BValue Saturation/1 -> B-Value/1
  [TankCooling] -> Sum3/1
  [Leakage] -> PerSec2PerCycle4/1
  Sum10/1 -> Sum8/1
  PerSec2PerCycle4/1 -> Sum10/2
  [TankMass] -> Sum8/2
  [InFlow1] -> Saturation2/1
  Saturation2/1 -> [SigInFlow1]
  [InFlow2] -> Saturation3/1
  Saturation3/1 -> [SigInFlow2]
  [InFlow3] -> Saturation4/1
  Saturation4/1 -> [SigInFlow3]
  Inlet1/3 -> [BasePressIn1]
  Inlet2/3 -> [BasePressIn2]
  Outlet2/3 -> [BasePressOut2]
  Outlet1/3 -> [BasePressOut1]
  Closed Position/1 -> Relational Operator3/2
  [Error] -> Relational Operator3/1
  [InFlowMass] -> Sum10/1
  Relational Operator3/1 -> Switch3/2
  Sum7/1 -> Switch3/3
  Switch3/1 -> [InFlowMass]
  Constant/1 -> Switch3/1
  Constant1/1 -> Mux3/6  "SinkAvailable"
  Constant3/1 -> Mux/6  "SinkAvailable"
  Constant4/1 -> Mux4/6  "SinkAvailable"
  Constant5/1 -> Mux5/6  "SinkAvailable"
  Demux4/6 -> Terminator11/1
  Demux5/6 -> Terminator12/1
  [Outlet1Height] -> Mux/8  "Height"
  Constant10/1 -> Mux/7  "VentAvailable"
  Demux4/7 -> Terminator14/1
  Demux4/8 -> Terminator13/1
  [Inlet1Height] -> Mux3/8  "Height"
  Constant11/1 -> Mux3/7  "VentAvailable"
  [Inlet2Height] -> Mux4/8  "Height"
  Constant12/1 -> Mux4/7  "VentAvailable"
  Demux5/7 -> Terminator18/1
  Demux5/8 -> Terminator17/1
  [Outlet2Height] -> Mux5/8  "Height"
  Constant13/1 -> Mux5/7  "VentAvailable"
  Side/1 -> [Side]
  Roll/1 -> [Roll]
  Level-2 MATLAB S-Function/2 -> [Probe2]
  [Probe2] -> Probe2/1
  [TankVolume] -> Level-2 MATLAB S-Function/3
  [Side] -> Level-2 MATLAB S-Function/1
  [Roll] -> Level-2 MATLAB S-Function/2
  Constant7/1 -> [Leakage]
  Constant18/1 -> [Outlet1Height]
  Constant19/1 -> [Inlet1Height]
  Constant20/1 -> [Outlet2Height]
  Constant21/1 -> [Inlet2Height]
  Constant22/1 -> [Inlet3Height]
  Constant23/1 -> [HeatConductance]
  Constant24/1 -> [SurfaceArea]
  Constant25/1 -> [AirTemp]
  Constant26/1 -> [ResetTemp]
  Constant27/1 -> [OverrideTemp]
  Constant28/1 -> [ResetMass]
  Constant29/1 -> [OverrideMass]
  Constant30/1 -> [ResetAValue]
  Constant31/1 -> [OverrideAValue]
  Constant32/1 -> [ResetBValue]
  Constant33/1 -> [OverrideBValue]
  Level-2 MATLAB S-Function/3 -> [SurfaceHeight]
  Level-2 MATLAB S-Function/4 -> [MaxVolume]
  Constant34/1 -> [Error]
  [TankInFlow] -> Terminator/1

== system FuelSystemLibrary/Temp2Density ==
  note: K-1
  note: Temperature2Density - implements the following formulae:
      |  - (K-1) = B - 0.00146T
      |  - (K-1) = D(A + 0.3568(K-1))
      |
      | Revision History -
      | Issue 1.0 - ?? - SW - Initial Issue
      | Issue 1.1 - 28th October 2005 - DR - Added to FSP Generic Library
  note: Avoid div-by-0
      | errors
  Temp : Inport
  AValue : Inport  Port=2
  BValue : Inport  Port=3
  Constant : Constant
  Constant1 : Constant
  Constant3 : Constant  Value=0.00146
  Constant4 : Constant  Value=0.3568
  Correct Units : Gain  Gain=kpl2kpm3  SaturateOnIntegerOverflow=on  OutDataTypeStr=Inherit: Same as input  ParamDataTypeStr=Inherit: Same as input
  ETZero : FuelSystemLibrary/ETZero
  ETZero1 : FuelSystemLibrary/ETZero
  Product1 : Product  Inputs=**  SaturateOnIntegerOverflow=on  InputSameDT=on  OutDataTypeStr=Inherit: Same as first input
  Product2 : Product  Inputs=**  SaturateOnIntegerOverflow=on  InputSameDT=on  OutDataTypeStr=Inherit: Same as first input
  Product3 : Product  Inputs=*/  SaturateOnIntegerOverflow=on  InputSameDT=on  OutDataTypeStr=Inherit: Same as first input
  Sum2 : Sum  Inputs=|+-  SaturateOnIntegerOverflow=on  InputSameDT=on  OutDataTypeStr=Inherit: Same as first input
  Sum3 : Sum  Inputs=|++  SaturateOnIntegerOverflow=on  InputSameDT=on  OutDataTypeStr=Inherit: Same as first input
  Switch : Switch  Threshold=BoolThreshold  SaturateOnIntegerOverflow=on  InputSameDT=on
  Switch1 : Switch  Threshold=BoolThreshold  SaturateOnIntegerOverflow=on  InputSameDT=on
  Density : Outport
  wires:
  [BValue] -> Sum2/1
  Product1/1 -> Sum2/2
  Temp/1 -> Product1/1
  Constant3/1 -> Product1/2
  Sum2/1 -> Product2/1, Switch1/3, ETZero1/1
  Constant4/1 -> Product2/2
  Product2/1 -> Sum3/1
  [AValue] -> Sum3/2
  Product3/1 -> Correct Units/1
  Correct Units/1 -> Density/1
  AValue/1 -> [AValue]
  BValue/1 -> [BValue]
  ETZero/1 -> Switch/2
  Constant/1 -> Switch/1
  Sum3/1 -> ETZero/1, Switch/3
  Switch/1 -> Product3/2
  Switch1/1 -> Product3/1
  ETZero1/1 -> Switch1/2
  Constant1/1 -> Switch1/1

== system FuelSystemLibrary/Temp2Dielectric ==
  note: Temperature2Dielectric - implements the following formulae:
      |  - (K-1) = B - 0.00146T
      |
      | Revision History -
      | Issue 1.0 - 11th October 2012 - SW - Initial Issue
  note: K-1
  Temp : Inport
  BValue : Inport  Port=2
  Constant : Constant
  Constant3 : Constant  Value=0.00146
  Product1 : Product  Inputs=**  SaturateOnIntegerOverflow=on  InputSameDT=on  OutDataTypeStr=Inherit: Same as first input
  Sum2 : Sum  Inputs=|+-  SaturateOnIntegerOverflow=on  InputSameDT=on  OutDataTypeStr=Inherit: Same as first input
  Sum3 : Sum  Inputs=|++  SaturateOnIntegerOverflow=on  InputSameDT=on  OutDataTypeStr=Inherit: Same as first input
  K : Outport
  wires:
  BValue/1 -> Sum2/1
  Sum2/1 -> Sum3/1
  Constant3/1 -> Product1/2
  Temp/1 -> Product1/1
  Product1/1 -> Sum2/2
  Sum3/1 -> K/1
  Constant/1 -> Sum3/2

== system FuelSystemLibrary/Valve1Ip ==
  En : Inport
  Valve2Ip : FuelSystemLibrary/Valve2Ip
  ValveIp : FuelSystemLibrary/ValveIp
  1P : PMIOPort  Tag=PMCPort  Port=1  Side=Left
  1BB : PMIOPort  Tag=PMCPort  Port=2  Side=Left
  2P : PMIOPort  Tag=PMCPort  Port=3  Side=Right
  2BB : PMIOPort  Tag=PMCPort  Port=4  Side=Right
  Open : Outport
  Shut : Outport  Port=2
  wires:
  En/1 -> ValveIp/1
  ValveIp/1 -> Valve2Ip/1
  Valve2Ip/1 -> Open/1
  Valve2Ip/2 -> Shut/1
  connections:
  Valve2Ip/RConn2 -- 2BB/RConn1
  Valve2Ip/RConn1 -- 2P/RConn1
  1BB/RConn1 -- Valve2Ip/LConn2
  1P/RConn1 -- Valve2Ip/LConn1

== system FuelSystemLibrary/Valve2Ip ==
  note: Valve is modelled by
      | variable resistance
  En : Inport
  BBBrk : FuelSystemLibrary/BBBrk
  BBBrk1 : FuelSystemLibrary/BBBrk1
  Constant2 : Constant  Value=InfiniteResistance
  Constant3 : Constant  Value=ValveOnResistance
  Demux1 : Demux  Outputs=8
  Demux2 : Demux  Outputs=8
  Enable{,1..5} (6 alike) : FuelSystemLibrary/Enable
  Mux2 : Mux  Inputs=8
  Mux3 : Mux  Inputs=8
  Product : Product  Inputs=*/  RndMeth=Zero
  Res : WrightSolverLib/Res
  Switch : Switch  Criteria=u2 ~= 0  SaturateOnIntegerOverflow=on
  ValveHead1 : Subsystem  RTWFcnName=ValveHead
      settings: RTWFcnNameOpts=User specified
  1P : PMIOPort  Tag=PMCPort  Port=1  Side=Left
  1BB : PMIOPort  Tag=PMCPort  Port=2  Side=Left
  2P : PMIOPort  Tag=PMCPort  Port=3  Side=Right
  2BB : PMIOPort  Tag=PMCPort  Port=4  Side=Right
  Open : Outport
  Shut : Outport  Port=2
  wires:
  BBBrk1/1 -> Demux2/1
  Mux3/1 -> BBBrk/1
  BBBrk/1 -> Demux1/1
  Mux2/1 -> BBBrk1/1
  Demux2/1 -> Mux3/1  "BasePress"
  Demux2/2 -> Mux3/2  "Temp"
  Demux2/3 -> Mux3/3  "AValue"
  Demux2/4 -> Mux3/4  "BValue"
  [ValveConducting] -> Enable/2
  Enable/1 -> Mux3/5
  Demux2/5 -> Enable/1  "SrcAvailable"
  [ValveConducting] -> Enable1/2
  Demux2/6 -> Enable1/1  "SinkAvailable"
  Enable1/1 -> Mux3/6
  Demux2/8 -> Mux3/8  "Height"
  Enable2/1 -> Mux3/7
  [ValveConducting] -> Enable2/2
  Demux2/7 -> Enable2/1  "VentAvailable"
  [ValveConducting] -> Enable3/2
  Demux1/5 -> Enable3/1  "SrcAvailable"
  [ValveConducting] -> Enable4/2
  Demux1/6 -> Enable4/1  "SinkAvailable"
  [ValveConducting] -> Enable5/2
  En/1 -> ValveHead1/1(En)
  Demux1/1 -> Mux2/1  "BasePress"
  Demux1/2 -> Mux2/2  "Temp"
  Demux1/3 -> Mux2/3  "AValue"
  Demux1/4 -> Mux2/4  "BValue"
  Enable3/1 -> Mux2/5
  Enable4/1 -> Mux2/6
  Demux1/7 -> Enable5/1  "VentAvailable"
  Enable5/1 -> Mux2/7
  Demux1/8 -> Mux2/8  "Height"
  Res/1 -> ValveHead1/2(Flow)  "Flow"
  ValveHead1/1(Open) -> Open/1
  Switch/1 -> Res/1
  Constant2/1 -> Switch/3
  [ValveConducting] -> Switch/2
  Product/1 -> Switch/1
  Constant3/1 -> Product/1
  ValveHead1/4(Conducting) -> [ValveConducting]
  ValveHead1/2(Shut) -> Shut/1
  ValveHead1/3(Pos) -> [Position]
  [Position] -> Product/2
  connections:
  1BB/RConn1 -- BBBrk1/RConn1
  Res/RConn1 -- 2P/RConn1
  1P/RConn1 -- Res/LConn1
  BBBrk/LConn1 -- 2BB/RConn1

== system FuelSystemLibrary/ValveEn ==
  note: ValveEn - Sets the Valve to constantly Enabled
      |
      | Revision History -
      | Issue 1.0  - ?? - SW - Initial Issue
      | Issue 1.1 - 28th October 2005 - DR - Added to FSP Generic Library
  Constant : Constant  Value=DiscreteSwitchOn
  Constant1 : Constant  Value=DiscreteSwitchOff
  Constant2 : Constant  Value=0
  Constant3 : Constant  Value=NoError
  Mux : Mux
  En : Outport
  wires:
  Mux/1 -> En/1
  Constant/1 -> Mux/1  "OnEn"
  Constant1/1 -> Mux/2  "OffEn"
  Constant2/1 -> Mux/3  "SwitchTime"
  Constant3/1 -> Mux/4  "ErrorCode"

== system FuelSystemLibrary/ValveIp ==
  note: Front-end to convert single input valve to 2-input
  1In : Inport
  Constant : Constant  Value=ValveOpenTime
  Constant1 : Constant  Value=NoError
  Data Type Conversion : DataTypeConversion  OutDataTypeStr=double
  Data Type Conversion1 : DataTypeConversion  OutDataTypeStr=double
  Data Type Conversion2 : DataTypeConversion  OutDataTypeStr=boolean
  Logical Operator : Logic  Operator=NOT
  Mux : Mux  Inputs=[1 1 1 1]
  2Out : Outport
  wires:
  Mux/1 -> 2Out/1
  Logical Operator/1 -> Data Type Conversion/1
  Constant/1 -> Mux/3
  Constant1/1 -> Mux/4
  1In/1 -> Data Type Conversion2/1
  Data Type Conversion/1 -> Mux/2
  Data Type Conversion1/1 -> Mux/1
  Data Type Conversion2/1 -> Logical Operator/1, Data Type Conversion1/1

== system FuelSystemLibrary/ValveStatStub ==
  note: ValveStatStub - used in congunction with ValveEn to suppress Valve status
      |
      | Revision History -
      | Issue 1.0 - ?? - SW - Initial Issue
      | Issue 1.1 - 28th October 2005 - DR - Added to FSP Generic Library
  Nul : Inport
  Terminator1 : Terminator
  wires:
  Nul/1 -> Terminator1/1

== system FuelSystemLibrary/ZeroOrderIntegrator ==
  note: ZeroOrderIntegrator
      |
      | Revision History -
      | Issue 1.0 - ?? - SW - Initial Issue
      | Issue 1.1 - 28th October 2005 - DR - Added to FSP Generic Library
  Inc : Inport
  PerSec2PerCycle : Gain  Gain=PerSec2PerCycle  OutDataTypeStr=Inherit: Same as input  ParamDataTypeStr=Inherit: Same as input
  Saturation : Saturate  UpperLimit=DiscreteSwitchOn  LowerLimit=DiscreteSwitchOff
  Sum : Sum  Inputs=|++  SaturateOnIntegerOverflow=on
  Unit Delay : UnitDelay  InitialCondition=DiscreteSwitchOff  SampleTime=-1
  Pos : Outport
  wires:
  Inc/1 -> PerSec2PerCycle/1
  Unit Delay/1 -> Pos/1, Sum/2
  Saturation/1 -> Unit Delay/1
  Sum/1 -> Saturation/1
  PerSec2PerCycle/1 -> Sum/1

== system FuelSystemLibrary/Bowser/FuelMeter ==
  note: Flow summing mechanism, with reset
      |
      | Uses crude rectangular integrator, for
      | commonality with Tank summing system
  RefuelReset : Inport
  DefuelReset : Inport  Port=2
  DefuelMeter : FuelSystemLibrary/Meter
  I Tap : WrightSolverLib/I Tap
  Ignore negative 2 : Saturate  UpperLimit=InfiniteFlow  LowerLimit=0
  Ignore negative1 : Saturate  UpperLimit=InfiniteFlow  LowerLimit=0
  Invert : Gain  Gain=-1  OutDataTypeStr=Inherit: Same as input  ParamDataTypeStr=Inherit: Same as input
  RefuelMeter : FuelSystemLibrary/Meter
  1P : PMIOPort  Tag=PMCPort  Port=1  Side=Left
  2P : PMIOPort  Tag=PMCPort  Port=2  Side=Right
  RefuelSum : Outport
  DefuelSum : Outport  Port=2
  wires:
  RefuelMeter/1 -> RefuelSum/1
  DefuelMeter/1 -> DefuelSum/1
  RefuelReset/1 -> RefuelMeter/1
  DefuelReset/1 -> DefuelMeter/1
  Ignore negative1/1 -> RefuelMeter/2
  Ignore negative 2/1 -> DefuelMeter/2
  I Tap/1 -> Ignore negative1/1, Invert/1
  Invert/1 -> Ignore negative 2/1
  connections:
  I Tap/RConn1 -- 2P/RConn1
  1P/RConn1 -- I Tap/LConn1

== system FuelSystemLibrary/Bowser/Subsystem4 ==
  1 : Inport
  2 : Inport  Port=2
  Terminator : Terminator
  Terminator1 : Terminator
  wires:
  1/1 -> Terminator/1
  2/1 -> Terminator1/1

== system FuelSystemLibrary/ParallelPumpPair/EnSplit1 ==
  En : Inport
  Demux2 : Demux  Outputs=9
  Terminator{1..2,4..7,13..14} (8 alike) : Terminator
  On : Outport
  wires:
  Demux2/9 -> Terminator13/1  "Flow"
  Demux2/6 -> Terminator4/1  "Mode"
  Demux2/3 -> Terminator7/1  "OnPress"
  Demux2/8 -> Terminator2/1  "Res"
  Demux2/5 -> Terminator5/1  "Error"
  Demux2/4 -> Terminator6/1  "OffPress"
  Demux2/2 -> Terminator14/1  "SwTime"
  Demux2/1 -> On/1  "On"
  Demux2/7 -> Terminator1/1  "Press"
  En/1 -> Demux2/1

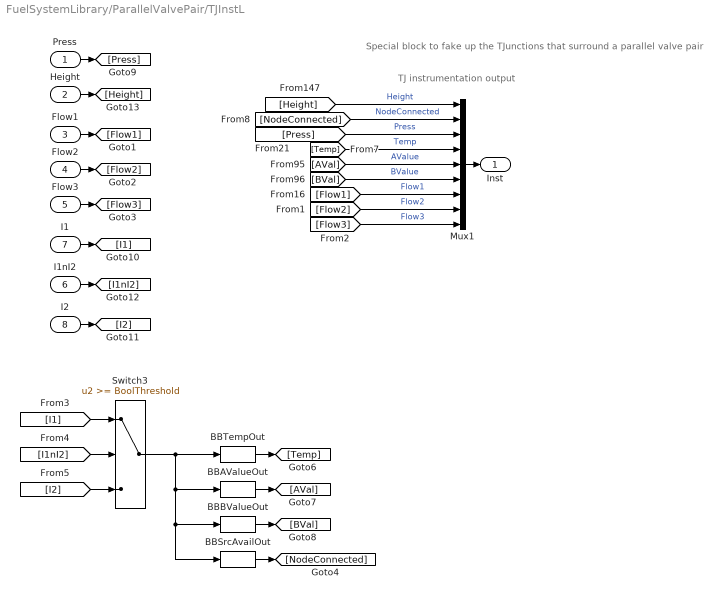
== system FuelSystemLibrary/ParallelValvePair/TJInstL ==
  note: Special block to fake up the TJunctions that surround a parallel valve pair
  note: TJ instrumentation
      |  output
  Press : Inport
  Height : Inport  Port=2
  Flow1 : Inport  Port=3
  Flow2 : Inport  Port=4
  Flow3 : Inport  Port=5
  I1nI2 : Inport  Port=6
  I1 : Inport  Port=7
  I2 : Inport  Port=8
  BBAValueOut : FuelSystemLibrary/BBAValueOut
  BBBValueOut : FuelSystemLibrary/BBBValueOut
  BBSrcAvailOut : FuelSystemLibrary/BBSrcAvailOut
  BBTempOut : FuelSystemLibrary/BBTempOut
  Mux1 : Mux  Inputs=9
  Switch3 : Switch  Threshold=BoolThreshold  SaturateOnIntegerOverflow=on  InputSameDT=on
  Inst : Outport
  wires:
  Height/1 -> [Height]
  [Height] -> Mux1/1  "Height"
  Mux1/1 -> Inst/1
  [BVal] -> Mux1/6  "BValue"
  [AVal] -> Mux1/5  "AValue"
  [Temp] -> Mux1/4  "Temp"
  [Press] -> Mux1/3  "Press"
  [Flow3] -> Mux1/9  "Flow3"
  [NodeConnected] -> Mux1/2  "NodeConnected"
  [Flow1] -> Mux1/7  "Flow1"
  [Flow2] -> Mux1/8  "Flow2"
  Flow1/1 -> [Flow1]
  Flow2/1 -> [Flow2]
  Flow3/1 -> [Flow3]
  Switch3/1 -> BBTempOut/1, BBAValueOut/1, BBBValueOut/1, BBSrcAvailOut/1
  BBTempOut/1 -> [Temp]
  BBAValueOut/1 -> [AVal]
  BBBValueOut/1 -> [BVal]
  Press/1 -> [Press]
  [I1nI2] -> Switch3/2
  I1/1 -> [I1]
  I2/1 -> [I2]
  BBSrcAvailOut/1 -> [NodeConnected]
  I1nI2/1 -> [I1nI2]
  [I1] -> Switch3/1
  [I2] -> Switch3/3

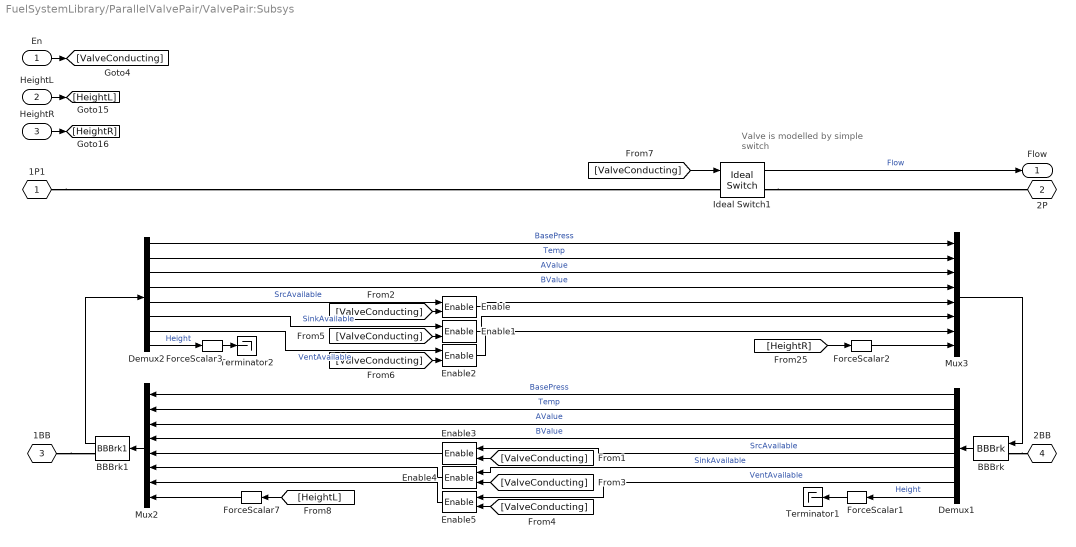
== system FuelSystemLibrary/ParallelValvePair/ValvePair:Subsys ==
  note: Valve is modelled by
      | simple switch
  En : Inport
  HeightL : Inport  Port=2
  HeightR : Inport  Port=3
  BBBrk : FuelSystemLibrary/BBBrk
  BBBrk1 : FuelSystemLibrary/BBBrk1
  Demux1 : Demux  Outputs=8
  Demux2 : Demux  Outputs=8
  Enable{,1..5} (6 alike) : FuelSystemLibrary/Enable
  ForceScalar{1..3,7} (4 alike) : FuelSystemLibrary/ForceScalar  SystemSampleTime=-1
  Ideal Switch1 : WrightSolverLib/Ideal Switch  OnResistance=ValveOnResistance
  Mux2 : Mux  Inputs=8
  Mux3 : Mux  Inputs=8
  Terminator1 : Terminator
  Terminator2 : Terminator
  1P1 : PMIOPort  Tag=PMCPort  Port=1  Side=Left
  2P : PMIOPort  Tag=PMCPort  Port=2  Side=Right
  1BB : PMIOPort  Tag=PMCPort  Port=3  Side=Left
  2BB : PMIOPort  Tag=PMCPort  Port=4  Side=Right
  Flow : Outport
  wires:
  ForceScalar1/1 -> Terminator1/1
  ForceScalar7/1 -> Mux2/8
  Demux1/8 -> ForceScalar1/1  "Height"
  [HeightL] -> ForceScalar7/1
  Enable5/1 -> Mux2/7
  Demux1/7 -> Enable5/1  "VentAvailable"
  Enable4/1 -> Mux2/6
  Enable3/1 -> Mux2/5
  Demux1/4 -> Mux2/4  "BValue"
  Demux1/3 -> Mux2/3  "AValue"
  Demux1/2 -> Mux2/2  "Temp"
  Demux1/1 -> Mux2/1  "BasePress"
  [ValveConducting] -> Enable5/2
  Demux1/6 -> Enable4/1  "SinkAvailable"
  [ValveConducting] -> Enable4/2
  Demux1/5 -> Enable3/1  "SrcAvailable"
  [ValveConducting] -> Enable3/2
  Demux2/7 -> Enable2/1  "VentAvailable"
  [ValveConducting] -> Enable2/2
  Enable2/1 -> Mux3/7
  Enable1/1 -> Mux3/6
  Demux2/6 -> Enable1/1  "SinkAvailable"
  [ValveConducting] -> Enable1/2
  Demux2/5 -> Enable/1  "SrcAvailable"
  Enable/1 -> Mux3/5
  [ValveConducting] -> Enable/2
  Demux2/4 -> Mux3/4  "BValue"
  Demux2/3 -> Mux3/3  "AValue"
  Demux2/2 -> Mux3/2  "Temp"
  Demux2/1 -> Mux3/1  "BasePress"
  Mux2/1 -> BBBrk1/1
  BBBrk/1 -> Demux1/1
  Mux3/1 -> BBBrk/1
  BBBrk1/1 -> Demux2/1
  [ValveConducting] -> Ideal Switch1/1
  En/1 -> [ValveConducting]
  Ideal Switch1/1 -> Flow/1  "Flow"
  HeightL/1 -> [HeightL]
  HeightR/1 -> [HeightR]
  [HeightR] -> ForceScalar2/1
  ForceScalar2/1 -> Mux3/8
  ForceScalar3/1 -> Terminator2/1
  Demux2/8 -> ForceScalar3/1  "Height"
  connections:
  BBBrk/LConn1 -- 2BB/RConn1
  1BB/RConn1 -- BBBrk1/RConn1
  Ideal Switch1/RConn1 -- 2P/RConn1
  1P1/RConn1 -- Ideal Switch1/LConn1
